simulink model "POWER_SYSTEM_FULL"  (R2025a)
settings: Solver=ode23t  StartTime=0  StopTime=5  FixedStep=1e-06  MinStep=1e-06  AbsTol=1e-6
model workspace (MAT data in the model file):
  CONTROL_INI : object (value not decoded)
  MODEL_INI : object (value not decoded)
  initialMemoryState = [1.15301991484 1.15301991484 1.15301991484 1.15301991484 0.612188611368 0.612188611368 0.612188611368 0.612188611368 -1.07438763375 -1.07438763375 -1.0821166602 -1.0821166602 ... (40 elements, 40x1)]
symbols that are objects in the model workspace (value not decoded): CONTROL_INI, MODEL_INI
undefined symbols (not defined in the file or in its folder): CONTROL, MODEL, monitorDFIG, pref_mask_vec, qref_mask_vec
(part 3 of 3)

== matlab function POWER_SYSTEM_FULL/CONTROL ==
  settings: updateMethod=CONTINUOUS  sampleTime=MODEL_INI.PARAM.SIM_SAMPLING_TIME
  data: STATE input; INPUT input size=10*MODEL_INI.DFIG.PARAM.nDFIG +1; CONTROL_IN input Bus: CONTROL_Bus; MODEL input Bus: MODEL_Bus; STATE_DERIVATIVE output; OUTPUT output size=4*MODEL_INI.DFIG.PARAM.nDFIG; CONTROL output Bus: CONTROL_Bus; t_OUT output; s_OUT output; d_IN input size=[7,MODEL_INI.DFIG.PARAM.nDFIG]; P_ref_IN input; Q_ref_IN input; breaker_status input size=[1,4]
function [STATE_DERIVATIVE,OUTPUT,CONTROL,t_OUT,s_OUT] = CONTROL_VSM(STATE,INPUT,CONTROL_IN,MODEL,d_IN,P_ref_IN,Q_ref_IN,breaker_status)

%% COPY CONTROL_BUS & MODEL_BUS
CONTROL = CONTROL_IN;
nDFIG = 4;

%--------------------------------------------------------------------------
%% PARAMETERS
%--------------------------------------------------------------------------
% Rated frequency
f0 = MODEL.BASE.f0;
w0 = 2*pi*f0;
%--------------------------------------------------------------------------
% DFIG PARAMETERS 
%--------------------------------------------------------------------------
% Induction machime parameters
ls = MODEL.DFIG.PARAM.Lsig_s_pu;
lr = MODEL.DFIG.PARAM.Lsig_r_pu;
Lm = MODEL.DFIG.PARAM.Lm_pu;
Ls = Lm + ls;
Lr = Lm + lr;
sg = 1 - Lm.^2./Ls./Lr;
% GSC filter reactance
Lfg = MODEL.DFIG.PARAM.Lfgsc_pu;
%--------------------------------------------------------------------------
% VSMP control parameters
%--------------------------------------------------------------------------
% Inertia [s]
H = CONTROL.VSMP.PARAM.H; 
% Steady-state damping
Dp = CONTROL.VSMP.PARAM.Dp; 
% Transient damping
Dd = CONTROL.VSMP.PARAM.Dd;
% VSMP derivative to error
der2error = CONTROL.VSMP.PARAM.der2error;
%--------------------------------------------------------------------------
% VSMQ control parameters
%--------------------------------------------------------------------------
% Voltage control
K_Fs_ref = CONTROL.VSMQ.PARAM.K_Fs_ref;
K_droopQV = CONTROL.VSMQ.PARAM.K_droopQV;
%--------------------------------------------------------------------------
% Virtual impedance
%--------------------------------------------------------------------------
Lv = CONTROL.VIMP.PARAM.Lv_pu;
% Rv = CONTROL.VIMP.PARAM.Rv_pu;
%--------------------------------------------------------------------------
% RSC current control (axid d) - Reactive power
%--------------------------------------------------------------------------
Kp_ird = CONTROL.RSCd.PARAM.Kp; 
Ki_ird = CONTROL.RSCd.PARAM.Ki; 
b_ird = CONTROL.RSCd.PARAM.b;  
%--------------------------------------------------------------------------
% RSC current control (axid q) - Active power
%--------------------------------------------------------------------------
Kp_irq = CONTROL.RSCq.PARAM.Kp; 
Ki_irq = CONTROL.RSCq.PARAM.Ki; 
b_irq = CONTROL.RSCq.PARAM.b;
%--------------------------------------------------------------------------
% DC-Link voltage control
%--------------------------------------------------------------------------
Kp_vdc = CONTROL.VDC.PARAM.Kp;
Ki_vdc = CONTROL.VDC.PARAM.Ki;
b_vdc = CONTROL.VDC.PARAM.b;
%--------------------------------------------------------------------------
% GSC current control (axid d) - Reactive power
%--------------------------------------------------------------------------
Kp_igd = CONTROL.GSCd.PARAM.Kp; 
Ki_igd = CONTROL.GSCd.PARAM.Ki; 
b_igd = CONTROL.GSCd.PARAM.b;  
%--------------------------------------------------------------------------
% GSC current control (axid q) - Active power
%--------------------------------------------------------------------------
Kp_igq = CONTROL.GSCq.PARAM.Kp; 
Ki_igq = CONTROL.GSCq.PARAM.Ki; 
b_igq = CONTROL.GSCq.PARAM.b;
%--------------------------------------------------------------------------
% CONVERTER CURRENT LIMITING + ANTI-WINDUP  (Reviewer 1, point 2)
%--------------------------------------------------------------------------
% All quantities below are LOCAL CONSTANTS. They are deliberately NOT read
% from the MODEL / CONTROL buses: adding a bus field would change the bus
% definition and force bus regeneration, which project_config.json classifies
% as a dangerous structural modification ("Initialization failure").
%
% LIM_EN  Master enable.  0 = DISABLED (default), 1 = ARMED.
%         With LIM_EN = 0 every limited quantity is blended out algebraically
%         and this block reproduces the unlimited model BIT-FOR-BIT, so all
%         previously published linear results, eigenvalues and GA designs are
%         unchanged.  Set LIM_EN = 1 for fault-ride-through studies.
LIM_EN = 0;
%
% I_PU2MODEL  Base conversion, pu-on-Ib -> MODEL current units.  CRITICAL.
%         The ratings below are quoted in pu on Ib, but the reference signals
%         this limiter acts on are NOT in that base.  The model's power
%         expression is  S = v.*conj(i)/sqrt(3)  (a line-to-line voltage
%         normalisation, consistent with MODEL.BASE.Zb = sqrt(3)*Ub^2/Sb =
%         Ub/Ib), so
%               i_pu(on Ib) = |i|_model / sqrt(3).
%         Both ratings are therefore converted ONCE, here.
%         Verified against ANALYSIS/TIER0_CURRENT_HEADROOM_RESULTS.md: at the
%         optimisation operating point |i_r| is 1.7796 / 1.8370 model units,
%         i.e. 1.0275 / 1.0606 pu on Ib, reproducing that table exactly.
%         Omitting this factor makes the limiter clamp the machine hard in
%         normal operation -- the same failure mode as using the 30 % power
%         figure, reached through a different door.
I_PU2MODEL = sqrt(3);
%
% I_RSC_MAX  Rotor-side converter current-magnitude rating [pu on Ib],
%         STATOR-REFERRED.  Base: Ib = 1760 A phase rms, Ub = 690 V (l-l),
%         Sb = 2.1034 MVA.  Every current in this model is stator-referred,
%         so NO turns-ratio factor (n = 2070/690 = 3) is applied anywhere.
%         1.074 pu, from the benchmark machine (Abad et al. 2011, "Doubly Fed
%         Induction Machine" -- the 2 MW DFIM modelled here):
%           Fig. 3.29 gives K'rs = 0.30-0.42; the primed quantity is three
%           times smaller than the stator-referred one  ->  0.90-1.26 pu
%           independent hand check                     ->  0.95   pu
%           direct derivation at the model rated point ->  1.0742 pu
%         WARNING: the commonly quoted "~30 % converter" figure is a POWER
%         rating tied to the slip range, NOT a current rating.  Using 0.3 pu
%         here would be wrong by roughly 3x and would clamp the machine in
%         normal operation.
%         Utilisation at the optimisation operating point is 95.7 % (DFIG 1-2)
%         and 98.8 % (DFIG 3-4): the limiter is INACTIVE there, but with
%         essentially no steady-state margin, so it does engage on transients.
I_RSC_MAX = 1.074 * I_PU2MODEL;         % = 1.86022 model units
%
% I_GSC_MAX  Grid-side converter current-magnitude rating [pu on Ib].
%         0.34 pu, from Abad Fig. 1.70 (~600 A against ~2000 A stator);
%         the Table 10.1 power cross-check gives 0.275 pu.
%         Utilisation at the optimisation operating point is 29.7 %.
I_GSC_MAX = 0.34 * I_PU2MODEL;          % = 0.58890 model units
%
% KAW_FS, KAW_VDC  Back-calculation anti-windup gains [1/s] for the two
%         integrators that FEED the limited references: the VSMQ stator-flux
%         reference Fs_ref (state 3, sets the RSC d-axis reference) and the
%         DC-link integrator I_vdc (state 6, sets the GSC q-axis reference).
%         Both are set to w0, i.e. a back-calculation tracking time constant
%         of 1/w0 = 3.2 ms: fast against the flux and DC-link loops, and no
%         faster than the electrical dynamics already present, so no new
%         stiffness is introduced.  Purely algebraic -- NO new states.
KAW_FS  = w0;
KAW_VDC = w0;
%
% VS_FLOOR  Denominator floor for the GSC power-to-current reference map
%         igd* = -sqrt(3)*Qg_ref/Vs,  igq* = sqrt(3)*Pg_ref/Vs   [pu voltage].
%         This is a NUMERICAL GUARD, NOT a control feature, so it is
%         DELIBERATELY NOT gated on LIM_EN: an unguarded division belongs in
%         no version of the model.  Without it a deep sag makes the reference
%         singular as Vs -> 0 and the limiter cannot rescue it, because min /
%         max propagate Inf and NaN rather than clamping them.
%
%         Value: 0.10 pu.  Justification is that below this terminal voltage
%         the GSC cannot export meaningful power anyway, so the floor removes
%         a numerical singularity WITHOUT altering achievable behaviour:
%           - the reference saturates once |igq*| >= I_GSC_MAX, i.e. once
%             |Pg_ref| >= Vs * 0.34 pu.  At Vs = VS_FLOOR that threshold is
%             only |Pg_ref| >= 0.034 pu, and during a sag the DC-link PI
%             drives |Pg_ref| to the trapped rotor power, of order 0.2-0.3 pu
%             -- an order of magnitude above it.  So for every condition in
%             which the floor is active the limiter is ALREADY clamping, and
%             the emitted reference is I_GSC_MAX either way.
%           - at the operating point Vs ~ 0.975 pu, so Vs_safe == Vs exactly
%             and the floor is inert.  Every published small-signal result is
%             therefore unchanged; this is verified, not asserted, by the
%             zero-difference regression with LIM_EN both 0 and 1.
%         0.05-0.20 pu is the conventional band.  0.10 pu is chosen rather
%         than 0.05 pu because the guard must sit ABOVE the deepest retained
%         voltage being studied (~0.05 pu), not at it: the failure being
%         removed is Vs UNDERSHOOTING during the transient, so a floor equal
%         to the retained voltage would still admit a 20x reference and would
%         only catch an exact zero crossing.
VS_FLOOR = 0.10;
%--------------------------------------------------------------------------
% RSC BLOCKING / DERATE -- FAULT-RIDE-THROUGH, SWITCHED, DEFAULT OFF
%--------------------------------------------------------------------------
% RSCBLK_EN  Master enable.  0 = DISABLED (default), 1 = ARMED, consistent
%         with LIM_EN and CHOP_EN.  With RSCBLK_EN = 0 the derate factor is
%         algebraically exactly 1 and every term it touches reduces to the
%         previous expression bit-for-bit, so the model reproduces the
%         no-blocking behaviour and the small-signal regression is untouched.
%
%         WHAT IT IS FOR -- the MEASURED root cause of the deep-sag DC-link
%         collapse.  In a deep sag the stator power collapses (-0.7383 ->
%         -0.0204 pu), so there is NO slip power left for the RSC to trap.
%         The RSC nevertheless keeps trying to regulate: it FLIPS P_RSC
%         POSITIVE (+0.5741 pu), pushing INTO the rotor to hold |ir| at the
%         limiter value against a collapsed flux, while the GSC still
%         exports.  The DC link drains and, without the Task-1 diode clamp,
%         goes NEGATIVE (-0.5825 pu).  The diode clamp BOUNDS that
%         consequence; this switch removes its CAUSE.
%
%         WHAT IT IS NOT.  It is NOT a latching crowbar.  A crowbar shorts
%         the rotor through a resistor and LATCHES until an explicit release
%         condition -- latching is by definition STATEFUL, and the standing
%         constraint here is NO NEW STATES.  This is the deliberately
%         lightweight option: the voltage-dependent DERATE of the rotor
%         voltage command that reproduces the part of a crowbar's effect
%         that matters for the DC link -- the RSC stops trying to regulate --
%         without the latch, without the rotor short, and without a state.
RSCBLK_EN = 0;
%
% VDCBLK_LO / VDCBLK_HI  DC-LINK-voltage blend band [pu on Udc_base].
%         *** THE TRIGGER IS Vdc, NOT THE TERMINAL VOLTAGE Vs. ***
%
%         WHY NOT Vs -- MEASURED, and the reason this was re-keyed.  A derate
%         keyed on the machine TERMINAL voltage closes a POSITIVE feedback
%         loop through the machine: blocking the RSC removes the DFIG's
%         excitation (the RSC is what magnetises a DFIG through the rotor),
%         so Vs falls FURTHER, which deepens the derate, which suppresses Vs
%         further.  It LATCHES with no state at all, because the loop closes
%         through the PLANT rather than through memory.  Measured at
%         r_src = 0.05 with the Vs-keyed band: at t = 0.36 s, 10 ms AFTER the
%         fault had cleared, Vs was 0.1719 and k_rsc was still 0.0000; at
%         t = 0.55 s, 200 ms after clearance, k_rsc was STILL 0.0000 and the
%         DC link sat at 0.0505 pu and never returned.  Avoiding a stateful
%         latch in the code did not avoid a latching mechanism in the plant.
%
%         Keying on Vdc INVERTS THE FEEDBACK SIGN and makes the derate
%         SELF-RELEASING: the RSC drains the link -> Vdc falls -> the derate
%         engages -> the drain stops -> Vdc recovers -> the derate releases.
%         No latch, no state, no hysteresis, no new signal.
%
%         AND IT IS THE STRONGER PHYSICAL STATEMENT.  A Vs-keyed derate is a
%         protection heuristic bolted onto the model.  A Vdc-keyed derate is
%         THE CONVERTER'S ACTUAL VOLTAGE CAPABILITY -- the one thing this
%         averaged model otherwise ignores, since it imposes vr EXACTLY as
%         commanded regardless of whether the DC link can synthesise it.
%         It is a modelling improvement that happens to have an FRT benefit,
%         rather than an FRT device.
%
%         THE BAND IS DERIVED, NOT PICKED, and the derivation is already in
%         the VDC_FLOOR block of the DFIG chart one chart over.  With SVPWM a
%         two-level bridge synthesises at most Vdc/sqrt(2) of line-to-line
%         RMS AC voltage, so the converter capability, in pu on the ROTOR
%         base (Ur_open_rotor_V = 2070 V), is the straight line
%
%             V_cap(Vdc) = Vdc * Udc_base/(sqrt(2)*Ur_open_rotor_V)
%                        = Vdc * 1200/(sqrt(2)*2070)
%                        = 0.409917 * Vdc          [pu on the rotor base]
%
%         (check: V_cap(0.50) = 0.204958 pu, which is the 0.205 pu the
%         VDC_FLOOR block quotes.)  BOTH band edges are that ONE line
%         evaluated against the TWO rotor-voltage demands the same block
%         already quantifies.  Neither edge is tuned; neither edge is round.
%
%         VDCBLK_LO -- capability = the IRREDUCIBLE BACK-EMF.
%           E_r = |s|*|Fs|*Lm/Ls = 0.1575228 * 1 * 2.0033344/2.0730505
%               = 0.152225 pu
%           at the pre-fault slip, and it GROWS as the rotor accelerates
%           during the fault.  |s| is READ from the stored operating point
%           (DFIG state 5, ROTOR SPEED = 1.1575228 -> s = -0.1575228), not
%           assumed.  Solving V_cap(Vdc) = E_r:
%               VDCBLK_LO = 0.152225/0.409917 = 0.371357 pu
%           BELOW THIS THE BRIDGE CANNOT SYNTHESISE EVEN THE MACHINE'S OWN
%           BACK-EMF.  There is no rotor voltage left to command at all; the
%           averaged model's core assumption -- vr imposed exactly as
%           commanded -- is not approximately false there, it is
%           definitively false.  The derate is COMPLETE at and below it.
%
%         VDCBLK_HI -- capability = the FULL DESIGN-SLIP rotor voltage.
%           The link is sized for the +-0.30 design slip, |vr| = 0.30 pu on
%           the rotor base (= 621 V).  Solving V_cap(Vdc) = 0.30:
%               VDCBLK_HI = 0.30/0.409917 = 0.731856 pu
%           which is the same 0.73 pu the VDC_FLOOR block already quotes
%           ("|vr| = 0.30*2070 = 621 V needs Vdc >= sqrt(2)*621 = 878 V =
%           0.73 pu"), here COMPUTED rather than rounded.  AT AND ABOVE THIS
%           THE CONVERTER HAS ITS FULL DESIGN AUTHORITY, so the command is
%           passed through untouched.
%
%         WHAT THE BAND INTERIOR MEANS, stated honestly as a modelling
%         choice.  Between the edges the converter retains PARTIAL
%         authority: at Vdc = 0.50 pu it can still synthesise 0.204958 pu,
%         more than the back-EMF and less than the design demand.  The exact
%         statement of that is a MAGNITUDE SATURATION of |vRSC| at
%         V_cap(Vdc).  A saturation is a hard kink in a state -- precisely
%         what the DC-link diode clamp next door was written to avoid -- and
%         it would put a non-smooth |.| of the command inside the
%         linearisation path.  The smoothstep is a deliberately CONSERVATIVE
%         C1 PROXY: monotone in Vdc, EXACT at both edges (full authority
%         above HI, none below LO), and it UNDER-states the retained
%         authority in between rather than over-stating it.
%
%         ONE DIFFERENCE FROM THE Vs-KEYED BAND IT REPLACES, recorded
%         because it matters for the paper: this band DOES engage inside the
%         region already valid under criterion (b).  It must -- it is a
%         CAPABILITY statement, not a protection threshold, and the
%         capability shortfall is real there.  It is mild: at the shallowest
%         sag of the V1 campaign (Vdc min 0.6705 pu) the blend is s = 0.8298
%         and k_rsc = 0.9230, i.e. 7.7 % suppression, released as Vdc
%         recovers.
%
%         INACTIVE AT THE OPERATING POINT -- VERIFIED, NOT ASSUMED.  DFIG
%         state 6 (DC VOLTAGE) reads EXACTLY 1 in the stored opModel of both
%         LIN_MODEL_FRD_OPT and LIN_MODEL_VI_OPT, for all four machines.
%         That is 0.268144 pu above VDCBLK_HI = 0.743813 band-widths, so the
%         ramp argument is saturated at 1 and k_rsc is not merely EQUAL to
%         1: its derivative with respect to Vdc is also EXACTLY 0, four
%         orders of magnitude beyond the 1e-5 NumericalPertRel step.
VDCBLK_LO = 0.371357;
VDCBLK_HI = 0.731856;
%
% KAW_RSC  Back-calculation anti-windup gain [1/s] for the two RSC
%         CURRENT-LOOP integrators I_ird and I_irq.  Set to w0, matching
%         KAW_FS and KAW_VDC: a tracking time constant of 1/w0 = 3.2 ms.
%         See the anti-windup block further down for why these two
%         integrators need a back-calculation path that they did NOT need
%         before this switch existed.
KAW_RSC = w0;

%--------------------------------------------------------------------------
%% STATE
%--------------------------------------------------------------------------
% VSMP
%--------------------------------------------------------------------------
x_VSMP = STATE(1,:);
th_VSMP = STATE(2,:);
%--------------------------------------------------------------------------
% VSMQ
%--------------------------------------------------------------------------
Fs_ref = STATE(3,:);
%--------------------------------------------------------------------------
% RSC
%--------------------------------------------------------------------------
I_ird = STATE(4,:);
I_irq = STATE(5,:);
%--------------------------------------------------------------------------
% VDC
%--------------------------------------------------------------------------
I_vdc = STATE(6,:);
%--------------------------------------------------------------------------
% GSC
%--------------------------------------------------------------------------
I_igd = STATE(7,:);
I_igq = STATE(8,:);

%--------------------------------------------------------------------------
%% INPUT
%--------------------------------------------------------------------------
% INPUT = [itr ; iti ; isr ; isi ; irr ; iri ; vsr ; vsi ; Vdc ; wr ; w]
itr = INPUT(0*nDFIG + (1:nDFIG))';
iti = INPUT(1*nDFIG + (1:nDFIG))';
isr = INPUT(2*nDFIG + (1:nDFIG))';
isi = INPUT(3*nDFIG + (1:nDFIG))';
irr = INPUT(4*nDFIG + (1:nDFIG))';
iri = INPUT(5*nDFIG + (1:nDFIG))';
vsr = INPUT(6*nDFIG + (1:nDFIG))';
vsi = INPUT(7*nDFIG + (1:nDFIG))';
Vdc = INPUT(8*nDFIG + (1:nDFIG))';
wr  = INPUT(9*nDFIG + (1:nDFIG))';
w   = INPUT(10*nDFIG + 1);
%--------------------------------------------------------------------------
% Stator voltage magnitude
%--------------------------------------------------------------------------
Vs_ref = CONTROL.VSMQ.TARGET.Vs_ref;
vs = vsr + 1j*vsi;
Vs = abs(vs);
CONTROL.VSMQ.INPUT.Vs = Vs;
%--------------------------------------------------------------------------
% DFIG reactive power
%--------------------------------------------------------------------------
Q_ref = CONTROL.VSMQ.TARGET.Q_ref + Q_ref_IN;
it = itr + 1j*iti;
is = isr + 1j*isi;
Q = imag(vs.*conj(it))/sqrt(3);
CONTROL.VSMQ.INPUT.Q = Q;
%--------------------------------------------------------------------------
% RSC current reference
%--------------------------------------------------------------------------
it_dq = it.*exp(-1j*th_VSMP);
is_dq = is.*exp(-1j*th_VSMP);
irdq_ref = 1./Lm.*(Fs_ref - Lv.*it_dq - Ls.*is_dq);
iRSCd_ref_raw = real(irdq_ref);
iRSCq_ref_raw = imag(irdq_ref);
%--------------------------------------------------------------------------
% RSC current-reference magnitude limiting -- d-AXIS PRIORITY
%--------------------------------------------------------------------------
% Frame convention of this model:  Fs_ref is REAL, i.e. the stator flux is
% aligned with the d-axis of the VSM frame (see the derivation below, which
% assumes Fsq = 0).  With flux on d:
%     Fsd = Lm*ird + Ls*isd   -> ird sets the MAGNETISING flux  -> voltage /
%                                reactive support
%     Te ~ Fsd*isq  and  Fsq = 0 = Lm*irq + Ls*isq  ->  irq ~ -Te  -> torque /
%                                active power
% So d = reactive, q = active in this frame, and the grid-code rule during a
% voltage sag -- reactive current first, active power curtailed -- is exactly
% d-axis priority.  Rule applied:
%     ird* is clamped to +-I_RSC_MAX;
%     irq* is then clamped to whatever is left on the rating circle,
%     +-sqrt(I_RSC_MAX^2 - ird*^2), which is 0 once d saturates.
% Note this is a deliberate modelling choice: a deep sag drives ird* to the
% rating and therefore curtails active power to zero for the duration of the
% fault.  That is the intended fault-ride-through behaviour, not a defect.
% THE GSC DOES NOT FOLLOW THIS RULE.  It takes q-axis (DC-link) priority; the
% asymmetry is deliberate and is justified at the GSC limiter block below.
% The RSC is the converter that delivers terminal reactive support in a DFIG,
% so reactive-current-first belongs HERE and only here.
iRSCd_ref_lim = min(max(iRSCd_ref_raw,-I_RSC_MAX),I_RSC_MAX);
iRSCq_room    = sqrt(max(I_RSC_MAX.^2 - iRSCd_ref_lim.^2,0));
iRSCq_ref_lim = min(max(iRSCq_ref_raw,-iRSCq_room),iRSCq_room);
% Algebraic enable-blend.  No if/else: Simulink compile-time dimension
% analysis stays trivial (same convention as MF_003_LINE_GRID), and with
% LIM_EN = 0 this returns the raw references bit-for-bit.
iRSCd_ref = (1-LIM_EN).*iRSCd_ref_raw + LIM_EN.*iRSCd_ref_lim;
iRSCq_ref = (1-LIM_EN).*iRSCq_ref_raw + LIM_EN.*iRSCq_ref_lim;
% Reference excess actually removed by the limiter -- identically 0 when
% LIM_EN = 0.  Feeds the back-calculation anti-windup of Fs_ref below.
iRSCd_exc = iRSCd_ref_raw - iRSCd_ref;
CONTROL.RSCd.TARGET.iRSCd_ref = iRSCd_ref;
CONTROL.RSCq.TARGET.iRSCq_ref = iRSCq_ref;
%--------------------------------------------------------------------------
% RSC current measurement
%--------------------------------------------------------------------------
ir = irr + 1j*iri;
ir_dq = ir.*exp(-1j*th_VSMP);
iRSCd = real(ir_dq);
iRSCq = imag(ir_dq);
CONTROL.RSCd.INPUT.iRSCd = iRSCd;
CONTROL.RSCq.INPUT.iRSCq = iRSCq;
%--------------------------------------------------------------------------
% DFIG active power
%--------------------------------------------------------------------------
P_ref = CONTROL.VSMP.TARGET.P_ref + P_ref_IN;
P = real(vs.*conj(it))/sqrt(3);
CONTROL.VSMP.INPUT.P = P;
%--------------------------------------------------------------------------
% DC-Link voltage [pu]
%--------------------------------------------------------------------------
% Reference
Vdc2_ref = CONTROL.VDC.TARGET.Vdc2_ref;
% Measurement
Vdc2 = Vdc.^2;
CONTROL.VDC.INPUT.Vdc2 = Vdc2;
%--------------------------------------------------------------------------
% GSC current measurement
%--------------------------------------------------------------------------
ig = -(it + is);
ig_dq = ig.*exp(-1j*th_VSMP);
iGSCd = real(ig_dq);
iGSCq = imag(ig_dq);
CONTROL.GSCd.INPUT.iGSCd = iGSCd;
CONTROL.GSCq.INPUT.iGSCq = iGSCq;
%--------------------------------------------------------------------------
% Stator voltage in dq
%--------------------------------------------------------------------------
vs_dq = vs.*exp(-1j*th_VSMP);
vsd = real(vs_dq); 
vsq = imag(vs_dq);

%--------------------------------------------------------------------------
%% STATE DERIVATIVE
%--------------------------------------------------------------------------
% VSMP
%--------------------------------------------------------------------------
w_VSMP_e = x_VSMP + (Dd/2./H).*(P_ref - P);
w_VSMP_y = x_VSMP - (Dd/2./H).*P;
w_VSMP_pu = w_VSMP_e.*(der2error) + w_VSMP_y.*(1 - der2error);
dx_VSMP = 1./(2*H).*(P_ref - P - Dp.*(w_VSMP_pu - 1));
%--------------------------------------------------------------------------
% Perturbation for control analysis
w_aux1 = Dp.*w_VSMP_pu;
w_aux2 = d_IN(1,:) + w_aux1;
%--------------------------------------------------------------------------
dth_VSMP = w0*(1./Dp.*w_aux2 - w);
%--------------------------------------------------------------------------
% VSMQ
%--------------------------------------------------------------------------
dFs_ref_aux = w0.*K_Fs_ref.*(K_droopQV.*(Vs_ref-Vs) + Q_ref - Q);
%--------------------------------------------------------------------------
% BACK-CALCULATION ANTI-WINDUP on the stator-flux reference (state 3)
%--------------------------------------------------------------------------
% Fs_ref is the ONLY integrator upstream of the RSC d-axis reference:
%     ird* = (Fs_ref - Lv*itd - Ls*isd)/Lm
% (the q-axis reference is a pure feed-forward of measured currents and has
% no integrator behind it).  When ird* is clamped, Fs_ref would otherwise
% keep integrating the voltage/reactive error -- during a sag Vs < Vs_ref
% indefinitely -- and wind up without bound.  The excess reference current
% iRSCd_exc is mapped back to flux units through Lm and subtracted from the
% integrator input.  This is ALGEBRAIC: it modifies an existing derivative
% and adds NO state.  It is applied to dFs_ref_aux, i.e. BEFORE the d_IN
% injection point, so the identity s_OUT = d_IN + t_OUT used by the control
% analysis is preserved.  Identically zero when LIM_EN = 0.
dFs_ref_aux = dFs_ref_aux - KAW_FS.*Lm.*iRSCd_exc;
%--------------------------------------------------------------------------
% Perturbation for control analysis
dFs_ref = d_IN(2,:) + dFs_ref_aux;
%--------------------------------------------------------------------------
% RSC current control
%--------------------------------------------------------------------------
% vr = Rr*ir + 1/w0*dFr/dt  + j*(w-wr)*Fr
% Fs = Lm*ir + Ls*is -> is = (Fs - Lm*ir)/Ls
% Fr = Lr*ir + Lm*is -> Fr = Lr*ir + Lm*((Fs - Lm*ir)/Ls 
% Fr = Lr*(1-Lm^2/Ls/Lr)*ir + Lm/Ls*Fs = sg*Lr*ir + Lm/Ls*Fs
% vr = Rr*ir + sg*Lr/w0*dir/dt + j*(w-wr)*sg*Lr*ir + Lm/Ls/w0*dFs/dt + j*(w-wr)*Lm/Ls*Fs
% It is assumed that dFsdq/dt = 0
% j*(w-wr)*Lm/Ls*Fsdq = j*(w-wr)*Lm/Ls*Fsd = 0
% vrdq = Rr*irdq + sg*Lr/w0*dirdq/dt + j*(w-wr)*sg*Lr*irdq 
% Rr*irdq + sg*Lr/w0*dirdq/dt = mvrdq = vrdq - j*(w-wr)*sg*Lr*irdq 
% mvrdq = vrdq - j*(w-wr)*sg*Lr*irdq
% vrd = mvrd - (w-wr)*sg*Lr*irq
% vrq = mvrq + (w-wr)*sg*Lr*ird
% mvrd: manipulated variable in axis d 
% mvrq: manipulated variable in axis q
%--------------------------------------------------------------------------
% ANTI-WINDUP SCOPE -- why the four current-loop integrators are excluded
%--------------------------------------------------------------------------
% I_ird, I_irq, I_igd, I_igq integrate the error against the LIMITED
% references set above.  A limited reference is by construction achievable,
% so these errors return to zero and these integrators do not wind up.
% Adding a back-calculation term here would double-count the same excess
% already handled at Fs_ref / I_vdc and would corrupt the current loops.
% They would need anti-windup only if the CONVERTER VOLTAGE saturated,
% which is not modelled (see the crowbar / DC-chopper further work).
%--------------------------------------------------------------------------
% RSCd
%--------------------------------------------------------------------------
dI_ird = Ki_ird.*(iRSCd_ref - iRSCd);
mvrd_aux = Kp_ird.*(b_ird.*iRSCd_ref - iRSCd) + I_ird;
%--------------------------------------------------------------------------
% Perturbation for control analysis
mvrd = d_IN(3,:) + mvrd_aux;
vRSCd = mvrd - (w_VSMP_pu - wr).*sg.*Lr.*iRSCq;
%--------------------------------------------------------------------------
% RSCq
%--------------------------------------------------------------------------
dI_irq = Ki_irq.*(iRSCq_ref - iRSCq);
mvrq_aux = Kp_irq.*(b_irq.*iRSCq_ref - iRSCq) + I_irq;
%--------------------------------------------------------------------------
% Perturbation for control analysis
mvrq = d_IN(4,:) + mvrq_aux;
vRSCq = mvrq + (w_VSMP_pu - wr).*sg.*Lr.*iRSCd;
%--------------------------------------------------------------------------
% RSC BLOCKING / DERATE FACTOR  (see RSCBLK_EN above)
%--------------------------------------------------------------------------
% Smoothstep blend on the DC-LINK voltage Vdc -- the converter's own
% synthesis capability (see VDCBLK_LO / VDCBLK_HI above).  Vdc is a chart
% INPUT, read far above from INPUT(8*nDFIG + (1:nDFIG)), exactly as Vs was,
% so re-keying the trigger introduces NO new signal path and NO new
% algebraic loop.
%
% C1 -- zero slope at BOTH ends.  Zero slope at the UPPER end is what keeps
% this switch exactly invisible to the linearisation: at the operating point
% Vdc = 1 pu EXACTLY (DFIG state 6 of the stored opModel, all four machines)
% the ramp argument is already saturated at 1, so k_rsc is not merely EQUAL
% to 1, its derivative with respect to Vdc is also exactly 0, and no
% numericalpert step of order 1e-5 can see it.  Zero slope at the LOWER end
% means the command is released and re-applied without a corner -- and
% unlike the Vs-keyed version this one DOES release, because a falling Vdc
% engages the derate, which stops the RSC drain, which raises Vdc again.
s_rscblk = min(max((Vdc - VDCBLK_LO)./(VDCBLK_HI - VDCBLK_LO), 0), 1);
k_rscblk = s_rscblk.^2.*(3 - 2.*s_rscblk);
% Identically 1 when RSCBLK_EN = 0: (1-0) + 0*k = 1 exactly, in floating point
% as well as in algebra, so every expression below reduces bit-for-bit.
k_rsc    = (1-RSCBLK_EN) + RSCBLK_EN.*k_rscblk;
%--------------------------------------------------------------------------
% BACK-CALCULATION ANTI-WINDUP on the RSC CURRENT-LOOP integrators (states 4,5)
%--------------------------------------------------------------------------
% THIS IS REQUIRED BY THE DERATE AND WAS NOT REQUIRED BEFORE IT.  The
% ANTI-WINDUP SCOPE note above excludes I_ird, I_irq, I_igd and I_igq from
% back-calculation, and gives a correct reason: they integrate the error
% against an ALREADY-LIMITED current reference, which is by construction
% achievable, so the error returns to zero on its own.  That note ends with
% the exact condition that would overturn it -- "They would need anti-windup
% only if the CONVERTER VOLTAGE saturated, which is not modelled".
%
% The RSC derate IS converter-voltage saturation.  It multiplies the rotor
% voltage command by k_rsc < 1, so the commanded current is no longer
% deliverable, the loop is open, and the error (iRSCd_ref - iRSCd) does NOT
% return to zero.  Left alone, I_ird and I_irq would integrate a persistent
% error against a command that is being thrown away -- windup against a
% blocked command, and the deeper the sag the worse it gets.  The two GSC
% current integrators are NOT affected: the derate does not touch vGSC.
%
% The excess is the voltage actually WITHHELD on each axis, (1-k_rsc)*vRSC,
% subtracted from the integrator input in the same back-calculation form the
% chart already uses twice (Fs_ref and I_vdc).  ALGEBRAIC, adds NO state.
% dI_ird and dI_irq were formed above and are corrected here, because the
% correction needs vRSCd and vRSCq -- exactly the pattern used for dI_vdc,
% which is formed before the GSC limiter and corrected after it.
%
% RE-DERIVED FOR THE Vdc TRIGGER, not carried over.  The excess is fixed by
% HOW the derate is APPLIED, not by WHAT TRIGGERS it: the command is vRSC,
% the applied voltage is k_rsc*vRSC, so the WITHHELD voltage is exactly
% (1 - k_rsc)*vRSC on each axis for ANY k_rsc in [0,1], whatever its
% argument.  The application point is unchanged -- a scalar multiply on the
% assembled dq command -- so the back-calculation above is unchanged in form
% and remains exact.  THREE THINGS DID HAVE TO BE RE-CHECKED, and all three
% hold:
%   1. Vdc, like Vs, is a chart INPUT and not a chart output, so keying on
%      it creates NO algebraic loop through the correction.
%   2. The correction is still a CONTRACTION on the command it corrects: at
%      equilibrium Ki*(iref - i) = KAW_RSC*(1 - k_rsc)*vRSC, the standard
%      back-calculation fixed point, which does not involve the trigger.
%   3. The correction now REINFORCES the self-release instead of feeding a
%      latch.  It drives |vRSC| down, which reduces the RSC drain on the
%      link, which raises Vdc, which raises k_rsc.  Under the Vs trigger
%      the identical correction fed the positive feedback; under the Vdc
%      trigger it feeds the recovery.  Same algebra, opposite loop sign.
% Identically ZERO when RSCBLK_EN = 0, and also identically zero whenever
% Vdc >= VDCBLK_HI regardless of RSCBLK_EN, since (1 - k_rsc) = 0 exactly --
% which is the case AT THE OPERATING POINT, where Vdc = 1 pu exactly.
% Fs_ref (state 3) and I_vdc (state 6) keep their existing back-calculation
% paths unchanged: their outputs are a CURRENT reference and a POWER
% reference respectively, not the derated voltage, so the derate does not
% open either of those loops directly.
dI_ird = dI_ird - KAW_RSC.*(1 - k_rsc).*vRSCd;
dI_irq = dI_irq - KAW_RSC.*(1 - k_rsc).*vRSCq;
%--------------------------------------------------------------------------
% VDC
%--------------------------------------------------------------------------
dI_vdc = Ki_vdc.*(Vdc2_ref - Vdc2);
Pg_ref_aux = Kp_vdc.*(b_vdc.*Vdc2_ref - Vdc2) + I_vdc;
%--------------------------------------------------------------------------
% Perturbation for control analysis
Pg_ref = d_IN(5,:) + Pg_ref_aux;
%--------------------------------------------------------------------------
% GSC current reference
%--------------------------------------------------------------------------
% vs - vg = Rfg*ig + Lfg/w0*dig/dt + j*w*Lfg*ig
% Rfg*ig + Lfg/w0*dig/dt = mvgdq = -vgdq + vsdq - j*w*Lfg*ig
% mvgdq = -vgdq + vsdq - j*w*Lfg*ig
% vgd = -mvgd + vsd + w*Lfg*igq
% vgq = -mvgq + vsq - w*Lfg*igd
% mvgd: manipulated variable in axis d 
% mvgq: manipulated variable in axis q
Qg_ref = CONTROL.GSCd.TARGET.Qg_ref;
% Guarded denominator -- see VS_FLOOR above.  Vs = abs(vs) >= 0, so a single
% max() is sufficient and no sign handling is needed.  UNCONDITIONAL: this is
% not gated on LIM_EN.  Vs_safe is used for BOTH axes so that the d and q
% references stay on a common scaling and their vector magnitude remains the
% quantity the rating circle below is expressed in.
Vs_safe = max(Vs, VS_FLOOR);
iGSCd_ref_raw = -sqrt(3)*Qg_ref./Vs_safe;
iGSCq_ref_raw =  sqrt(3)*Pg_ref./Vs_safe;
%--------------------------------------------------------------------------
% GSC current-reference magnitude limiting -- q-AXIS PRIORITY (DC-LINK FIRST)
%--------------------------------------------------------------------------
% THE SPLIT BETWEEN THE TWO CONVERTERS IS ASYMMETRIC BY DESIGN, NOT BY
% OVERSIGHT.  The RSC keeps d-axis (reactive-current-first) priority; the GSC
% takes q-axis (DC-link-first) priority.  The reason is that the grid-code
% rule "reactive current first" is a requirement at the MACHINE TERMINALS,
% and in a DFIG that reactive support is delivered by the ROTOR-SIDE
% converter THROUGH THE STATOR.  The GSC's function is DC-link regulation;
% its reactive capability is secondary and, at 0.34 pu rating against the
% RSC's 1.074 pu, marginal in any case.  Giving the GSC's scarce rating to
% reactive current buys almost no terminal support while surrendering the
% one job only the GSC can do.
%
% This SUPERSEDES the earlier d-priority choice, which was applied to the GSC
% "for consistency with the RSC" and was contradicted by its own measurements:
% with d priority a deep sag squeezed the q-axis reference, the DC link went
% unregulated, Vdc reached 1.52 pu (against 1.24 pu UNLIMITED) and the actual
% GSC current still reached 0.439 pu against its 0.340 pu rating -- i.e. the
% limiter made both the DC-link excursion AND the current excursion WORSE
% than no limiter at all.  A limiter that degrades the quantity it exists to
% bound is misconfigured, not conservative.
%
% Rule applied:
%     igq* is clamped FIRST to +-I_GSC_MAX (full rating circle);
%     igd* is then bounded by whatever is left, +-sqrt(I_GSC_MAX^2 - igq*^2),
%     which is 0 once q saturates.
iGSCq_ref_lim = min(max(iGSCq_ref_raw,-I_GSC_MAX),I_GSC_MAX);
iGSCd_room    = sqrt(max(I_GSC_MAX.^2 - iGSCq_ref_lim.^2,0));
iGSCd_ref_lim = min(max(iGSCd_ref_raw,-iGSCd_room),iGSCd_room);
iGSCd_ref = (1-LIM_EN).*iGSCd_ref_raw + LIM_EN.*iGSCd_ref_lim;
iGSCq_ref = (1-LIM_EN).*iGSCq_ref_raw + LIM_EN.*iGSCq_ref_lim;
% Excess removed by the limiter -- identically 0 when LIM_EN = 0.
iGSCq_exc = iGSCq_ref_raw - iGSCq_ref;
%--------------------------------------------------------------------------
% BACK-CALCULATION ANTI-WINDUP on the DC-link integrator (state 6)
%--------------------------------------------------------------------------
% I_vdc is the integrator upstream of the GSC q-axis reference through
% Pg_ref -> igq* = sqrt(3)*Pg_ref/Vs_safe.  When igq* is clamped the DC-link
% error persists and I_vdc would wind up.  The current excess is converted
% back to power units and subtracted from the integrator input.  ALGEBRAIC,
% adds NO state.  dI_vdc was formed above; it is corrected here because the
% correction needs the GSC limiter result, and STATE_DERIVATIVE is assembled
% further below.
%
% RE-DERIVED for q-axis priority, not assumed to carry over.  The question is
% which integrator each clamped axis winds up, and the answer is unchanged:
%   - q carries Pg_ref, and Pg_ref IS the output of the DC-link integrator
%     I_vdc.  Clamping q therefore winds up I_vdc, and the excess that must
%     be back-calculated is the UNHONOURED q reference, iGSCq_ref_raw -
%     iGSCq_ref, which is exactly what iGSCq_exc computes.  The expression
%     below is therefore still correct with q clamped first.
%   - d carries Qg_ref, which is a CONSTANT TARGET read straight from
%     CONTROL.GSCd.TARGET.Qg_ref -- there is NO integrator behind igd*.  So
%     the newly-second axis needs no anti-windup of its own, and adding one
%     would have nothing to act on.
% What DOES change is the magnitude, not the structure: under d priority the
% q reference was squeezed by whatever d had taken, so iGSCq_exc was large
% whenever the sag was deep.  Under q priority q is clamped only against the
% full rating circle, so iGSCq_exc is nonzero strictly less often and is
% smaller when it is nonzero.  That is the intended effect.
%
% The back-calculation gain uses Vs_safe, NOT Vs, and this is deliberate.
% Back-calculation must invert the map that was ACTUALLY APPLIED.  The
% forward map is igq* = sqrt(3)*Pg_ref/Vs_safe, so its exact inverse is
% multiplication by Vs_safe/sqrt(3); that makes KAW_VDC*iGSCq_exc*Vs_safe/
% sqrt(3) precisely the power the limiter refused to honour.  Using the raw
% Vs would scale the correction by Vs/Vs_safe < 1 whenever the floor is
% active -- i.e. it would UNDER-correct the windup exactly in the deepest
% sags, where windup is worst, and would decay to zero as Vs -> 0, disabling
% the anti-windup at the very singularity the floor exists to remove.
% At the operating point Vs_safe == Vs, so this choice is invisible to the
% small-signal model (and iGSCq_exc is identically 0 when LIM_EN = 0).
dI_vdc = dI_vdc - KAW_VDC.*iGSCq_exc.*Vs_safe./sqrt(3);
CONTROL.GSCd.TARGET.iGSCd_ref = iGSCd_ref;
CONTROL.GSCq.TARGET.iGSCq_ref = iGSCq_ref;
%--------------------------------------------------------------------------
% GSCd
%--------------------------------------------------------------------------
dI_igd = Ki_igd.*(iGSCd_ref - iGSCd);
mvgd_aux = Kp_igd.*(b_igd.*iGSCd_ref - iGSCd) + I_igd;
%--------------------------------------------------------------------------
% Perturbation for control analysis
mvgd = d_IN(6,:) + mvgd_aux;
vGSCd = -mvgd + vsd + iGSCq.*w_VSMP_pu.*Lfg;
%--------------------------------------------------------------------------
% GSCq
%--------------------------------------------------------------------------
dI_igq = Ki_igq.*(iGSCq_ref - iGSCq);
mvgq_aux = Kp_igq.*(b_igq.*iGSCq_ref - iGSCq) + I_igq;
%--------------------------------------------------------------------------
% Perturbation for control analysis
mvgq = d_IN(7,:) + mvgq_aux;
vGSCq = -mvgq + vsq - iGSCd.*w_VSMP_pu.*Lfg;
%--------------------------------------------------------------------------
% State derivative
%--------------------------------------------------------------------------
STATE_DERIVATIVE = [dx_VSMP ; dth_VSMP ; dFs_ref ; dI_ird ; dI_irq ; ...
                    dI_vdc ; dI_igd ; dI_igq];

%--------------------------------------------------------------------------
% BREAKER LOGIC: freeze states of disconnected generators
%--------------------------------------------------------------------------
STATE_DERIVATIVE = STATE_DERIVATIVE .* breaker_status;

%--------------------------------------------------------------------------
%% OUTPUT 
%--------------------------------------------------------------------------
% VSMP
%--------------------------------------------------------------------------
CONTROL.VSMP.OUTPUT.w_pu = w_VSMP_pu;
CONTROL.VSMP.OUTPUT.dth = dth_VSMP;
CONTROL.VSMP.OUTPUT.th = th_VSMP;
CONTROL.VSMP.OUTPUT.MV = w_aux1;
%--------------------------------------------------------------------------
% VSMQ
%--------------------------------------------------------------------------
CONTROL.VSMQ.OUTPUT.Fs_ref = Fs_ref;
CONTROL.VSMQ.OUTPUT.MV = dFs_ref;
%--------------------------------------------------------------------------
% RSCd
%--------------------------------------------------------------------------
CONTROL.RSCd.OUTPUT.vRSCd = vRSCd;
CONTROL.RSCd.OUTPUT.MV = mvrd;
%--------------------------------------------------------------------------
% RSCq
%--------------------------------------------------------------------------
CONTROL.RSCq.OUTPUT.vRSCq = vRSCq;
CONTROL.RSCq.OUTPUT.MV = mvrq;
%--------------------------------------------------------------------------
% VDC
%--------------------------------------------------------------------------
CONTROL.VDC.OUTPUT.Pg_ref = Pg_ref;
CONTROL.VDC.OUTPUT.MV = Pg_ref;
%--------------------------------------------------------------------------
% GSCd
%--------------------------------------------------------------------------
CONTROL.GSCd.OUTPUT.vGSCd = vGSCd;
CONTROL.GSCd.OUTPUT.MV = mvgd;
%--------------------------------------------------------------------------
% GSCq
%--------------------------------------------------------------------------
CONTROL.GSCq.OUTPUT.vGSCq = vGSCq;
CONTROL.GSCq.OUTPUT.MV = mvgq;

%--------------------------------------------------------------------------
%% CONTROL ANALYSIS
%--------------------------------------------------------------------------
t_OUT = [w_aux1 ; dFs_ref_aux ; mvrd_aux ; mvrq_aux ; Pg_ref_aux ; mvgd_aux ; mvgq_aux];
s_OUT = [w_aux2 ; dFs_ref ; mvrd ; mvrq ; Pg_ref ; mvgd ; mvgq];

%--------------------------------------------------------------------------
%% STATE UPDATE
%--------------------------------------------------------------------------
CONTROL.VSMP.STATE = STATE(1:2,:);
CONTROL.VSMQ.STATE = STATE(3,:);
CONTROL.RSCd.STATE = STATE(4,:);
CONTROL.RSCq.STATE = STATE(5,:);
CONTROL.VDC.STATE = STATE(6,:);
CONTROL.GSCd.STATE = STATE(7,:);
CONTROL.GSCq.STATE = STATE(8,:);

%--------------------------------------------------------------------------
%% CONNECTIONS WITH THE POWER SYSTEM
%--------------------------------------------------------------------------
% RSC voltage
%--------------------------------------------------------------------------
% RSC BLOCKING / DERATE APPLIED (see RSCBLK_EN above).  Applied HERE, on the
% assembled dq command and downstream of every d_IN injection point, so the
% identities the control analysis relies on are preserved exactly.  Scaling
% by k_rsc is a rotation-invariant magnitude derate: it suppresses the
% command without altering its angle, which is what a blocked converter does
% -- it stops imposing a voltage, it does not impose a different one.
vRSC_dq = k_rsc.*(vRSCd + 1j*vRSCq);
vRSC_ri = vRSC_dq.*exp(1j*th_VSMP);
%--------------------------------------------------------------------------
% GSC voltage
%--------------------------------------------------------------------------
vGSC_dq = vGSCd + 1j*vGSCq;
vGSC_ri = vGSC_dq.*exp(1j*th_VSMP);
%--------------------------------------------------------------------------
% BREAKER LOGIC: zero control voltages of disconnected generators
%--------------------------------------------------------------------------
vRSC_ri = vRSC_ri .* breaker_status;
vGSC_ri = vGSC_ri .* breaker_status;

%--------------------------------------------------------------------------
% OUTPUT = [vrr ; vri ; vgr ; vgi]
%--------------------------------------------------------------------------
OUTPUT = zeros(4*nDFIG,1);
OUTPUT(0*nDFIG + (1:nDFIG)) = real(vRSC_ri(:));
OUTPUT(1*nDFIG + (1:nDFIG)) = imag(vRSC_ri(:));
OUTPUT(2*nDFIG + (1:nDFIG)) = real(vGSC_ri(:));
OUTPUT(3*nDFIG + (1:nDFIG)) = imag(vGSC_ri(:));

return
